simulink model "Model_2"  (R2017b)
settings: Solver=FixedStepAuto  StartTime=0.0  StopTime=inf  RelTol=1e-3  EnableMultiTasking=on
undefined symbols (not defined in the file or in its folder): nmea, sl_nmea
libraries: raspberrypilib x1
settings Model: SimulationMode=external  Creator=bb6223s  LastModifiedBy=bb6223s
settings SolverCC: PositivePriorityOrder=on
settings OptimizationCC: PassReuseOutputArgsAs=Individual arguments  MaxStackSize=64
settings DebuggingCC: ParameterTunabilityLossMsg=error
settings HardwareCC: ProdBitPerPointer=32  ProdBitPerSizeT=32  ProdBitPerPtrDiffT=32  ProdLargestAtomicInteger=Long  ProdLargestAtomicFloat=Double  ProdWordSize=32  ProdHWDeviceType=ARM Compatible->ARM Cortex
settings SFSimCC: SimUserIncludeDirs=U:\Navigation Project\Codes\ilsf-nmea-5564b320662e\tbx\NMEA Toolbox  MATLABDynamicMemAlloc=off
settings RTWCC: SystemTargetFile=ert.tlc  HardwareBoard=Raspberry Pi  TemplateMakefile=ert_default_tmf  GenerateReport=on  Toolchain=GNU GCC Raspberry Pi  IncludeHyperlinkInReport=on  LaunchReport=on  GenerateTraceInfo=on  GenerateTraceReport=on  GenerateTraceReportSl=on  GenerateTraceReportSf=on  GenerateTraceReportEml=on
settings CodeAppCC: ForceParamTrailComments=on  IgnoreCustomStorageClasses=off  OperatorAnnotations=on  SimulinkDataObjDesc=on  SFDataObjDesc=on  InsertBlockDesc=on
settings ERTTargetCC: SupportNonInlinedSFcns=on  SupportVariableSizeSignals=on
settings ConfigComp: PSAutoStubLUT=on

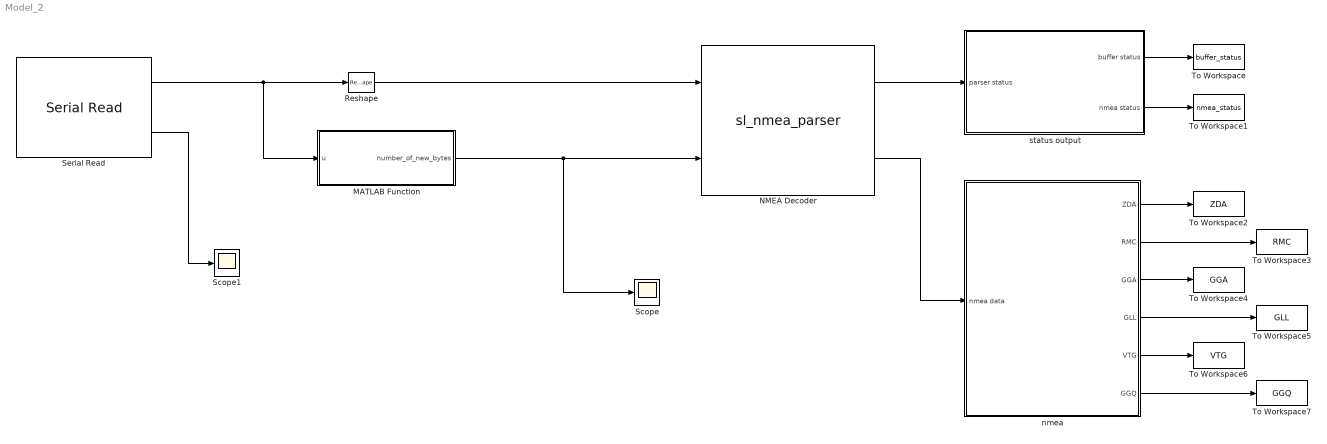
== system Model_2 ==
  MATLAB Function : MATLAB Function  TreatAsAtomicUnit=on
  NMEA Decoder : S-Function  AncestorBlock=sl_nmea/NMEA Decoder  FunctionName=sl_nmea_parser  SFunctionModules='nmea0183 circularbuffer'  SFunctionDeploymentMode=off  EnableBusSupport=off
  Reshape : Reshape
  Scope : Scope
  Scope1 : Scope
  Serial Read : raspberrypilib/Serial Read  board=Pi 3 Model B  SCIModule_=/dev/ttyACM0  Baudrate_=115200  Parity=None  StopBits_=1  HardwareFlowControl=None  ByteOrder=LittleEndian  DataLength=300  DataType=uint8  OutputStatus=on  SampleTime=0.1  blockPlatform=RaspberryPi
      settings: SourceProductName=Simulink Support Package for Raspberry Pi Hardware  SourceProductBaseCode=RASPPI
  To Workspace : ToWorkspace  VariableName=buffer_status  SaveFormat=Timeseries  SampleTime=-1
  To Workspace1 : ToWorkspace  VariableName=nmea_status  SaveFormat=Timeseries  SampleTime=-1
  To Workspace2 : ToWorkspace  VariableName=ZDA  SaveFormat=Timeseries  SampleTime=-1
  To Workspace3 : ToWorkspace  VariableName=RMC  SaveFormat=Timeseries  SampleTime=-1
  To Workspace4 : ToWorkspace  VariableName=GGA  SaveFormat=Timeseries  SampleTime=-1
  To Workspace5 : ToWorkspace  VariableName=GLL  SaveFormat=Timeseries  SampleTime=-1
  To Workspace6 : ToWorkspace  VariableName=VTG  SaveFormat=Timeseries  SampleTime=-1
  To Workspace7 : ToWorkspace  VariableName=GGQ  SaveFormat=Timeseries  SampleTime=-1
  nmea : Subsystem  AncestorBlock=sl_nmea/nmea
  status output : Subsystem  AncestorBlock=sl_nmea/status output
  wires:
  Serial Read/2 -> Scope1/1
  NMEA Decoder/1 -> status output/1(parser status)
  NMEA Decoder/2 -> nmea/1(nmea data)
  nmea/1(ZDA) -> To Workspace2/1
  nmea/2(RMC) -> To Workspace3/1
  nmea/3(GGA) -> To Workspace4/1
  nmea/4(GLL) -> To Workspace5/1
  nmea/5(VTG) -> To Workspace6/1
  nmea/6(GGQ) -> To Workspace7/1
  status output/1(buffer status) -> To Workspace/1
  status output/2(nmea status) -> To Workspace1/1
  Serial Read/1 -> Reshape/1, MATLAB Function/1(u)
  MATLAB Function/1(number_of_new_bytes) -> Scope/1, NMEA Decoder/2
  Reshape/1 -> NMEA Decoder/1

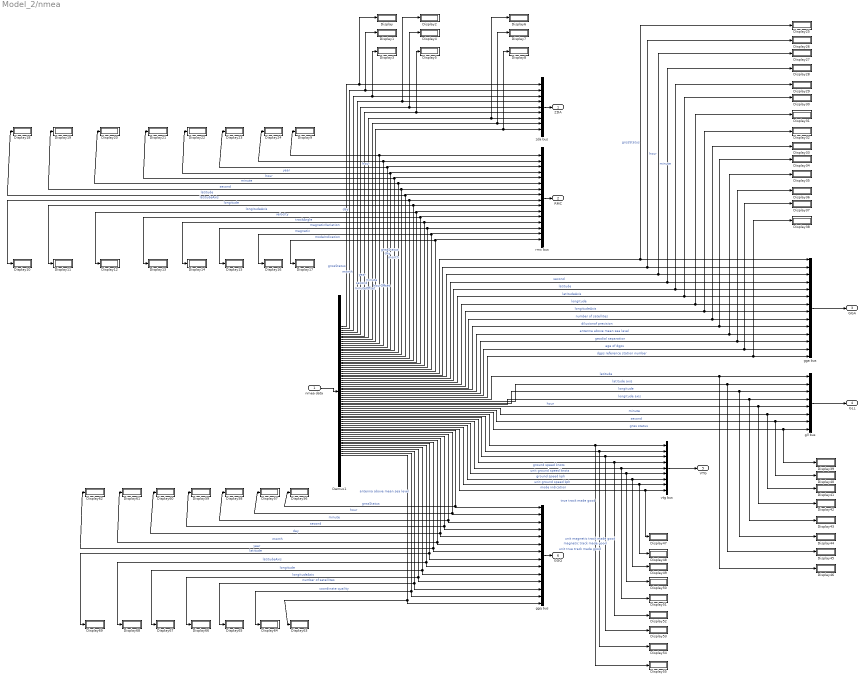
== system Model_2/nmea ==
  nmea data : Inport
  Demux1 : Demux  Outputs=70
  Display{,1..69} (70 alike) : Display
  gga bus : BusCreator  Inputs=14
  ggq bus : BusCreator  Inputs=14
  gll bus : BusCreator  Inputs=8
  rmc bus : BusCreator  Inputs=16
  vtg bus : BusCreator  Inputs=9
  zda bus : BusCreator  Inputs=9
  ZDA : Outport
  RMC : Outport  Port=2
  GGA : Outport  Port=3
  GLL : Outport  Port=4
  VTG : Outport  Port=5
  GGQ : Outport  Port=6
  wires:
  Demux1/1 -> Display/1, zda bus/1  "gnssStatus"
  nmea data/1 -> Demux1/1
  zda bus/1 -> ZDA/1
  Demux1/2 -> Display1/1, zda bus/2  "day"
  Demux1/3 -> Display3/1, zda bus/3  "month"
  Demux1/4 -> Display2/1, zda bus/4  "year"
  Demux1/5 -> Display4/1, zda bus/5  "hour"
  Demux1/6 -> Display5/1, zda bus/6  "minute"
  Demux1/7 -> Display6/1, zda bus/7  "second"
  Demux1/8 -> Display7/1, zda bus/8  "hourOffset"
  Demux1/9 -> Display8/1, zda bus/9  "minuteOffset"
  rmc bus/1 -> RMC/1
  Demux1/10 -> Display9/1, rmc bus/1  "gnssStatus"
  Demux1/11 -> Display24/1, rmc bus/2  "day"
  Demux1/12 -> Display23/1, rmc bus/3  "month"
  Demux1/13 -> Display22/1, rmc bus/4  "year"
  Demux1/14 -> Display21/1, rmc bus/5  "hour"
  Demux1/15 -> Display20/1, rmc bus/6  "minute"
  Demux1/16 -> Display19/1, rmc bus/7  "second"
  Demux1/17 -> Display18/1, rmc bus/8  "latitude"
  Demux1/18 -> Display10/1, rmc bus/9  "latitudeAxis"
  Demux1/19 -> Display11/1, rmc bus/10  "longitude"
  Demux1/20 -> Display12/1, rmc bus/11  "longitudeAxis"
  Demux1/21 -> Display13/1, rmc bus/12  "velocity"
  Demux1/22 -> Display14/1, rmc bus/13  "trackAngle"
  Demux1/23 -> Display15/1, rmc bus/14  "magneticVariation"
  Demux1/24 -> Display16/1, rmc bus/15  "magnetic"
  Demux1/25 -> Display17/1, rmc bus/16  "modeIndication"
  gga bus/1 -> GGA/1
  Demux1/26 -> Display25/1, gga bus/1  "gnssStatus"
  Demux1/27 -> Display26/1, gga bus/2  "hour"
  Demux1/28 -> Display27/1, gga bus/3  "minute"
  Demux1/29 -> Display28/1, gga bus/4  "second"
  Demux1/30 -> Display29/1, gga bus/5  "latitude"
  Demux1/31 -> Display30/1, gga bus/6  "latitudeAxis"
  Demux1/32 -> Display31/1, gga bus/7  "longitude"
  Demux1/33 -> Display32/1, gga bus/8  "longitudeAxis"
  Demux1/34 -> Display33/1, gga bus/9  "number of satellites"
  Demux1/35 -> Display34/1, gga bus/10  "dilusionof precision"
  Demux1/36 -> Display35/1, gga bus/11  "antenna above mean sea level"
  Demux1/37 -> Display36/1, gga bus/12  "geodial separation"
  Demux1/38 -> Display37/1, gga bus/13  "age of dgps"
  Demux1/39 -> Display38/1, gga bus/14  "dgps reference station number"
  gll bus/1 -> GLL/1
  vtg bus/1 -> VTG/1
  Demux1/40 -> Display46/1, gll bus/1  "latitude"
  Demux1/41 -> Display45/1, gll bus/2  "latitude axis"
  Demux1/42 -> Display44/1, gll bus/3  "longitude"
  Demux1/43 -> Display43/1, gll bus/4  "longitude axis"
  Demux1/44 -> Display42/1, gll bus/5  "hour"
  Demux1/45 -> Display41/1, gll bus/6  "minute"
  Demux1/46 -> Display40/1, gll bus/7  "second"
  Demux1/47 -> Display39/1, gll bus/8  "gnss status"
  Demux1/48 -> Display55/1, vtg bus/1  "true track made good"
  Demux1/49 -> Display54/1, vtg bus/2  "unit true track made good"
  Demux1/50 -> Display53/1, vtg bus/3  "magnetic track made good"
  Demux1/51 -> Display52/1, vtg bus/4  "unit magnetic track made good"
  Demux1/52 -> Display51/1, vtg bus/5  "ground speed knots"
  Demux1/53 -> Display50/1, vtg bus/6  "unit ground speed knots"
  Demux1/54 -> Display49/1, vtg bus/7  "ground speed kph"
  Demux1/55 -> Display48/1, vtg bus/8  "unit ground speed kph"
  Demux1/56 -> Display47/1, vtg bus/9  "mode indication"
  ggq bus/1 -> GGQ/1
  Demux1/57 -> Display56/1, ggq bus/1  "gnssStatus"
  Demux1/58 -> Display57/1, ggq bus/2  "hour"
  Demux1/59 -> Display58/1, ggq bus/3  "minute"
  Demux1/60 -> Display59/1, ggq bus/4  "second"
  Demux1/61 -> Display60/1, ggq bus/5  "day"
  Demux1/62 -> Display61/1, ggq bus/6  "month"
  Demux1/63 -> Display62/1, ggq bus/7  "year"
  Demux1/64 -> Display69/1, ggq bus/8  "latitude"
  Demux1/65 -> Display68/1, ggq bus/9  "latitudeAxis"
  Demux1/66 -> Display67/1, ggq bus/10  "longitude"
  Demux1/67 -> Display66/1, ggq bus/11  "longitudeAxis"
  Demux1/68 -> Display65/1, ggq bus/12  "number of satellites"
  Demux1/69 -> Display64/1, ggq bus/13  "coordinate quality"
  Demux1/70 -> Display63/1, ggq bus/14  "antenna above mean sea level"

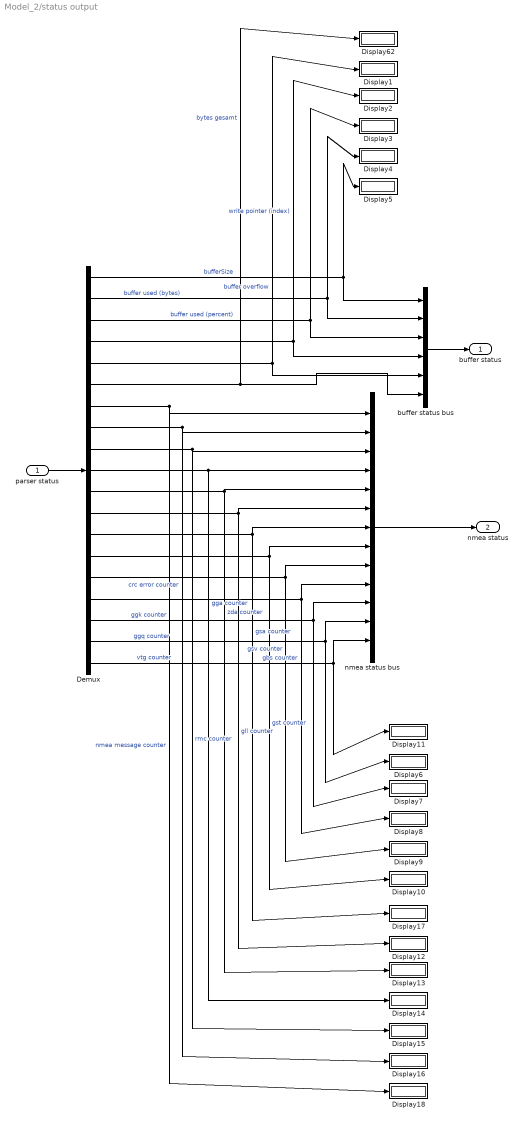
== system Model_2/status output ==
  parser status : Inport
  Demux : Demux  Outputs=19
  Display{1..18,62} (19 alike) : Display
  buffer status bus : BusCreator  Inputs=6
  nmea status bus : BusCreator  Inputs=13
  buffer status : Outport
  nmea status : Outport  Port=2
  wires:
  Demux/1 -> Display5/1, buffer status bus/1  "bufferSize"
  parser status/1 -> Demux/1
  Demux/2 -> Display4/1, buffer status bus/2  "buffer used (bytes)"
  Demux/3 -> Display3/1, buffer status bus/3  "buffer used (percent)"
  Demux/4 -> Display2/1, buffer status bus/4  "write pointer (index)"
  Demux/5 -> Display1/1, buffer status bus/5  "buffer overflow"
  Demux/6 -> Display62/1, buffer status bus/6  "bytes gesamt"
  Demux/7 -> Display18/1, nmea status bus/1  "nmea message counter"
  Demux/8 -> Display16/1, nmea status bus/2  "crc error counter"
  Demux/9 -> Display15/1, nmea status bus/3  "rmc counter"
  Demux/10 -> Display14/1, nmea status bus/4  "gga counter"
  Demux/11 -> Display13/1, nmea status bus/5  "zda counter"
  Demux/12 -> Display12/1, nmea status bus/6  "gll counter"
  Demux/13 -> Display17/1, nmea status bus/7  "gsa counter"
  Demux/14 -> Display10/1, nmea status bus/8  "gst counter"
  Demux/15 -> Display9/1, nmea status bus/9  "gsv counter"
  Demux/16 -> Display8/1, nmea status bus/10  "gbs counter"
  buffer status bus/1 -> buffer status/1
  nmea status bus/1 -> nmea status/1
  Demux/17 -> Display7/1, nmea status bus/11  "ggk counter"
  Demux/18 -> Display6/1, nmea status bus/12  "ggq counter"
  Demux/19 -> Display11/1, nmea status bus/13  "vtg counter"

== matlab function Model_2/MATLAB Function ==
  data: u input; number_of_new_bytes output uint32 size=1
function number_of_new_bytes = fcn(u)
% number_of_new_bytes = 1;
a=find(u>0,1,'last');
if isempty(a)
    a=0;
end
number_of_new_bytes = uint32(a(1));
